simulink model "P702_NI_SoftECU"  (R2019a)
settings: Solver=ode1  StartTime=0.0  StopTime=Inf  FixedStep=0.001  RelTol=1e-3  EnableMultiTasking=on
PreLoadFcn:
  | run '.\VeriStand_BlockSet\NIVeriStandAddPaths.m'
undefined symbols (not defined in the file or in its folder): magnitude
libraries: simulink x83, simulink_extras x1
(part 71 of 76)

== system P702_NI_SoftECU/SoftECU/SRR_R/RearRight_SOD/SRR_RR_002/Subsystem ==
  target_pos : Inport
  sensor_pos : Inport  Port=2
  CSP : Inport  Port=3
  Abs : Abs
  Add : Sum  Inputs=++-+
  Add1 : Sum  Inputs=++-+
  Add2 : Sum  Inputs=+-
  Add3 : Sum
  Bus Selector : BusSelector  OutputSignals=SRR_R_DET_RANGE_02[m],SRR_R_DET_AZIMUTH_02[rad],SRR_R_DET_RANGE_RATE_02[m/s],SRR_R_DET_ELEVATION_02[rad]
  Bus Selector1 : BusSelector  OutputSignals=sensor_x,sensor_y,sensor_yaw
  Bus Selector2 : BusSelector  OutputSignals=c_sensor_x,c_sensor_y,c_sensor_yaw
  Constant : Constant
  Index Vector : MultiPortSwitch  DataPortOrder=Zero-based contiguous  Inputs=2  zeroidx=on
  Index Vector1 : MultiPortSwitch  DataPortOrder=Zero-based contiguous  Inputs=2  zeroidx=on
  Logical Operator : Logic  AllPortsSameDT=off  OutDataTypeStr=boolean
  Math Function : Math  Operator=magnitude^2  SaturateOnIntegerOverflow=on
  Math Function1 : Math  Operator=magnitude^2  SaturateOnIntegerOverflow=on
  Product : Product
  Product1 : Product
  Product2 : Product
  Relational Operator : RelationalOperator  Operator=<=  OutDataTypeStr=boolean  RndMeth=Simplest
  Relational Operator1 : RelationalOperator  Operator=<=  OutDataTypeStr=boolean  RndMeth=Simplest
  Sqrt : Sqrt  SaturateOnIntegerOverflow=on
  Terminator : Terminator
  atan_cal : Trigonometry  Operator=atan2
  atan_cal1 : Trigonometry  Operator=atan2
  not_valid_azimuth : Constant  Value=0
  not_valid_range : Constant  Value=-1
  random_factor : Subsystem
  random_factor1 : Subsystem
  sincal : Trigonometry
  sincal1 : Trigonometry  Operator=cos
  sincal2 : Trigonometry
  sincal3 : Trigonometry  Operator=cos
  range : Outport
  range_rate : Outport  Port=2
  azimuth : Outport  Port=3
  elevation : Outport  Port=4
  wires:
  random_factor1/1(Rand_Error) -> Add1/4
  random_factor/1(Rand_Error) -> Add/4
  [AngleScanRange] -> Relational Operator1/2
  [DistanceScanRange] -> Relational Operator/2
  Abs/1 -> Relational Operator1/1
  Add2/1 -> sincal2/1, sincal3/1
  sincal3/1 -> atan_cal1/2
  sincal2/1 -> atan_cal1/1
  atan_cal1/1 -> Product2/1
  not_valid_azimuth/1 -> Index Vector1/2
  Logical Operator/1 -> Index Vector/1, Index Vector1/1
  Index Vector1/1 -> azimuth/1
  not_valid_range/1 -> Index Vector/2
  Index Vector/1 -> range/1
  Relational Operator1/1 -> Logical Operator/2
  Relational Operator/1 -> Logical Operator/1
  Product2/1 -> Index Vector1/3, Abs/1
  Sqrt/1 -> Relational Operator/1, Index Vector/3
  Bus Selector/4 -> elevation/1  "<SRR_R_DET_ELEVATION_02[rad]>"
  Bus Selector/3 -> range_rate/1  "<SRR_R_DET_RANGE_RATE_02[m/s]>"
  Constant/1 -> Product2/2
  Add3/1 -> Sqrt/1
  Math Function1/1 -> Add3/2
  Math Function/1 -> Add3/1
  atan_cal/1 -> Add2/1
  Add1/1 -> atan_cal/2, Math Function1/1
  Add/1 -> atan_cal/1, Math Function/1
  Product1/1 -> Add1/1
  Bus Selector1/3 -> Add2/2  "<sensor_yaw>"
  Bus Selector1/2 -> Add/3  "<sensor_y>"
  Bus Selector1/1 -> Add1/3  "<sensor_x>"
  Bus Selector2/3 -> Terminator/1  "<c_sensor_yaw>"
  Bus Selector2/2 -> Add/2  "<c_sensor_y>"
  Bus Selector2/1 -> Add1/2  "<c_sensor_x>"
  CSP/1 -> Bus Selector2/1
  sensor_pos/1 -> Bus Selector1/1
  Product/1 -> Add/1
  sincal1/1 -> Product1/2
  sincal/1 -> Product/2
  Bus Selector/2 -> sincal/1, sincal1/1  "<SRR_R_DET_AZIMUTH_02[rad]>"
  Bus Selector/1 -> Product/1, Product1/1, random_factor1/1(Range), random_factor/1(Range)  "<SRR_R_DET_RANGE_02[m]>"
  target_pos/1 -> Bus Selector/1

== system P702_NI_SoftECU/SoftECU/SRR_R/RearRight_SOD/SRR_RR_003/Subsystem ==
  target_pos : Inport
  sensor_pos : Inport  Port=2
  CSP : Inport  Port=3
  Abs : Abs
  Add : Sum  Inputs=++-+
  Add1 : Sum  Inputs=++-+
  Add2 : Sum  Inputs=+-
  Add3 : Sum
  Bus Selector : BusSelector  OutputSignals=SRR_R_DET_RANGE_03[m],SRR_R_DET_AZIMUTH_03[rad],SRR_R_DET_RANGE_RATE_03[m/s],SRR_R_DET_ELEVATION_03[rad]
  Bus Selector1 : BusSelector  OutputSignals=sensor_x,sensor_y,sensor_yaw
  Bus Selector2 : BusSelector  OutputSignals=c_sensor_x,c_sensor_y,c_sensor_yaw
  Constant : Constant
  Index Vector : MultiPortSwitch  DataPortOrder=Zero-based contiguous  Inputs=2  zeroidx=on
  Index Vector1 : MultiPortSwitch  DataPortOrder=Zero-based contiguous  Inputs=2  zeroidx=on
  Logical Operator : Logic  AllPortsSameDT=off  OutDataTypeStr=boolean
  Math Function : Math  Operator=magnitude^2  SaturateOnIntegerOverflow=on
  Math Function1 : Math  Operator=magnitude^2  SaturateOnIntegerOverflow=on
  Product : Product
  Product1 : Product
  Product2 : Product
  Relational Operator : RelationalOperator  Operator=<=  OutDataTypeStr=boolean  RndMeth=Simplest
  Relational Operator1 : RelationalOperator  Operator=<=  OutDataTypeStr=boolean  RndMeth=Simplest
  Sqrt : Sqrt  SaturateOnIntegerOverflow=on
  Terminator : Terminator
  atan_cal : Trigonometry  Operator=atan2
  atan_cal1 : Trigonometry  Operator=atan2
  not_valid_azimuth : Constant  Value=0
  not_valid_range : Constant  Value=-1
  random_factor : Subsystem
  random_factor1 : Subsystem
  sincal : Trigonometry
  sincal1 : Trigonometry  Operator=cos
  sincal2 : Trigonometry
  sincal3 : Trigonometry  Operator=cos
  range : Outport
  range_rate : Outport  Port=2
  azimuth : Outport  Port=3
  elevation : Outport  Port=4
  wires:
  target_pos/1 -> Bus Selector/1
  Bus Selector/1 -> random_factor/1(Range), random_factor1/1(Range), Product1/1, Product/1  "<SRR_R_DET_RANGE_03[m]>"
  Bus Selector/2 -> sincal1/1, sincal/1  "<SRR_R_DET_AZIMUTH_03[rad]>"
  sincal/1 -> Product/2
  sincal1/1 -> Product1/2
  Product/1 -> Add/1
  sensor_pos/1 -> Bus Selector1/1
  CSP/1 -> Bus Selector2/1
  Bus Selector2/1 -> Add1/2  "<c_sensor_x>"
  Bus Selector2/2 -> Add/2  "<c_sensor_y>"
  Bus Selector2/3 -> Terminator/1  "<c_sensor_yaw>"
  Bus Selector1/1 -> Add1/3  "<sensor_x>"
  Bus Selector1/2 -> Add/3  "<sensor_y>"
  Bus Selector1/3 -> Add2/2  "<sensor_yaw>"
  Product1/1 -> Add1/1
  Add/1 -> Math Function/1, atan_cal/1
  Add1/1 -> Math Function1/1, atan_cal/2
  atan_cal/1 -> Add2/1
  Math Function/1 -> Add3/1
  Math Function1/1 -> Add3/2
  Add3/1 -> Sqrt/1
  Constant/1 -> Product2/2
  Bus Selector/3 -> range_rate/1  "<SRR_R_DET_RANGE_RATE_03[m/s]>"
  Bus Selector/4 -> elevation/1  "<SRR_R_DET_ELEVATION_03[rad]>"
  Sqrt/1 -> Index Vector/3, Relational Operator/1
  Product2/1 -> Abs/1, Index Vector1/3
  Relational Operator/1 -> Logical Operator/1
  Relational Operator1/1 -> Logical Operator/2
  Index Vector/1 -> range/1
  not_valid_range/1 -> Index Vector/2
  Index Vector1/1 -> azimuth/1
  Logical Operator/1 -> Index Vector1/1, Index Vector/1
  not_valid_azimuth/1 -> Index Vector1/2
  atan_cal1/1 -> Product2/1
  sincal2/1 -> atan_cal1/1
  sincal3/1 -> atan_cal1/2
  Add2/1 -> sincal3/1, sincal2/1
  Abs/1 -> Relational Operator1/1
  [DistanceScanRange] -> Relational Operator/2
  [AngleScanRange] -> Relational Operator1/2
  random_factor/1(Rand_Error) -> Add/4
  random_factor1/1(Rand_Error) -> Add1/4

== system P702_NI_SoftECU/Output/Subsystem1/CAN_Signal/GWM/GSM/Gear_Shift_by_Wire_2_FD1_168 ==
  in_port : Inport
  GearButtnStuck_B_Actl : Terminator
  GsmSrvcRqd_B_Rq : Terminator
  TrnGearPwmFalt_B_Actl : Terminator
  TrnTrcmPwmSig_D_Actl : Terminator
  bus_selector : BusSelector  OutputSignals=GearButtnStuck_B_Actl,GsmSrvcRqd_B_Rq,TrnGearPwmFalt_B_Actl,TrnTrcmPwmSig_D_Actl
  wires:
  in_port/1 -> bus_selector/1  "Subsystem1"
  bus_selector/1 -> GearButtnStuck_B_Actl/1  "<GearButtnStuck_B_Actl>"
  bus_selector/2 -> GsmSrvcRqd_B_Rq/1  "<GsmSrvcRqd_B_Rq>"
  bus_selector/3 -> TrnGearPwmFalt_B_Actl/1  "<TrnGearPwmFalt_B_Actl>"
  bus_selector/4 -> TrnTrcmPwmSig_D_Actl/1  "<TrnTrcmPwmSig_D_Actl>"

== system P702_NI_SoftECU/Output/Subsystem1/CAN_Signal/GWM/GSM/Gear_Shift_by_Wire_FD1_5A ==
  in_port : Inport
  BrkSwtchPos_B_ActlGsm : Terminator
  DrQltyDrv_D_StatGsm : Terminator
  GsmGearMsgTxt_D_Rq : Terminator
  PrkBrkActv_D_RqGsmGear : Terminator
  TrnBtsiOvrrd_B_Stat : Terminator
  TrnGearButtn_B_ActlD0 : Terminator
  TrnGearButtn_B_ActlD1 : Terminator
  TrnGearButtn_B_ActlD2 : Terminator
  TrnGearButtn_B_ActlM0 : Terminator
  TrnGearButtn_B_ActlM1 : Terminator
  TrnGearButtn_B_ActlM2 : Terminator
  TrnGearButtn_B_ActlN0 : Terminator
  TrnGearButtn_B_ActlN1 : Terminator
  TrnGearButtn_B_ActlN2 : Terminator
  TrnGearButtn_B_ActlP0 : Terminator
  TrnGearButtn_B_ActlP1 : Terminator
  TrnGearButtn_B_ActlP2 : Terminator
  TrnGearButtn_B_ActlR0 : Terminator
  TrnGearButtn_B_ActlR1 : Terminator
  TrnGearButtn_B_ActlR2 : Terminator
  TrnGearButtn_U_Actl : Terminator
  TrnGearRqCnt_B_Actl : Terminator
  TrnGear_D_RqDrv : Terminator
  TrnGear_No_Cnt : Terminator
  TrnGear_No_Cs : Terminator
  TrnGsmNtmState_D_Actl : Terminator
  TrnRng_D_RqGsm : Terminator
  TrnValidGearRq_D_Stat : Terminator
  bus_selector : BusSelector  OutputSignals=BrkSwtchPos_B_ActlGsm,DrQltyDrv_D_StatGsm,GsmGearMsgTxt_D_Rq,PrkBrkActv_D_RqGsmGear,TrnBtsiOvrrd_B_Stat,TrnGearButtn_B_ActlD0,TrnGearButtn_B_ActlD1,TrnGearButtn_B_ActlD2,TrnGearButtn_B_ActlM0,TrnGearButtn_B_ActlM1,TrnGearButtn_B_ActlM2,TrnGearButtn_B_ActlN0,TrnGearButtn_B_ActlN1,TrnGearButtn_B_ActlN2,TrnGearButtn_B_ActlP0,TrnGearButtn_B_ActlP1,TrnGearButtn_B_ActlP2,TrnGearButtn_B_ActlR0,TrnGearButtn_B_ActlR1,TrnGearButtn_B_ActlR2,TrnGearButtn_U_Actl,TrnGearRqCnt_B_Actl,TrnGear_D_RqDrv,TrnGear_No_Cnt,TrnGear_No_Cs,TrnGsmNtmState_D_Actl,TrnRng_D_RqGsm,TrnValidGearRq_D_Stat
  wires:
  in_port/1 -> bus_selector/1  "Subsystem1"
  bus_selector/1 -> BrkSwtchPos_B_ActlGsm/1  "<BrkSwtchPos_B_ActlGsm>"
  bus_selector/2 -> DrQltyDrv_D_StatGsm/1  "<DrQltyDrv_D_StatGsm>"
  bus_selector/3 -> GsmGearMsgTxt_D_Rq/1  "<GsmGearMsgTxt_D_Rq>"
  bus_selector/4 -> PrkBrkActv_D_RqGsmGear/1  "<PrkBrkActv_D_RqGsmGear>"
  bus_selector/5 -> TrnBtsiOvrrd_B_Stat/1  "<TrnBtsiOvrrd_B_Stat>"
  bus_selector/6 -> TrnGearButtn_B_ActlD0/1  "<TrnGearButtn_B_ActlD0>"
  bus_selector/7 -> TrnGearButtn_B_ActlD1/1  "<TrnGearButtn_B_ActlD1>"
  bus_selector/8 -> TrnGearButtn_B_ActlD2/1  "<TrnGearButtn_B_ActlD2>"
  bus_selector/9 -> TrnGearButtn_B_ActlM0/1  "<TrnGearButtn_B_ActlM0>"
  bus_selector/10 -> TrnGearButtn_B_ActlM1/1  "<TrnGearButtn_B_ActlM1>"
  bus_selector/11 -> TrnGearButtn_B_ActlM2/1  "<TrnGearButtn_B_ActlM2>"
  bus_selector/12 -> TrnGearButtn_B_ActlN0/1  "<TrnGearButtn_B_ActlN0>"
  bus_selector/13 -> TrnGearButtn_B_ActlN1/1  "<TrnGearButtn_B_ActlN1>"
  bus_selector/14 -> TrnGearButtn_B_ActlN2/1  "<TrnGearButtn_B_ActlN2>"
  bus_selector/15 -> TrnGearButtn_B_ActlP0/1  "<TrnGearButtn_B_ActlP0>"
  bus_selector/16 -> TrnGearButtn_B_ActlP1/1  "<TrnGearButtn_B_ActlP1>"
  bus_selector/17 -> TrnGearButtn_B_ActlP2/1  "<TrnGearButtn_B_ActlP2>"
  bus_selector/18 -> TrnGearButtn_B_ActlR0/1  "<TrnGearButtn_B_ActlR0>"
  bus_selector/19 -> TrnGearButtn_B_ActlR1/1  "<TrnGearButtn_B_ActlR1>"
  bus_selector/20 -> TrnGearButtn_B_ActlR2/1  "<TrnGearButtn_B_ActlR2>"
  bus_selector/21 -> TrnGearButtn_U_Actl/1  "<TrnGearButtn_U_Actl>"
  bus_selector/22 -> TrnGearRqCnt_B_Actl/1  "<TrnGearRqCnt_B_Actl>"
  bus_selector/23 -> TrnGear_D_RqDrv/1  "<TrnGear_D_RqDrv>"
  bus_selector/24 -> TrnGear_No_Cnt/1  "<TrnGear_No_Cnt>"
  bus_selector/25 -> TrnGear_No_Cs/1  "<TrnGear_No_Cs>"
  bus_selector/26 -> TrnGsmNtmState_D_Actl/1  "<TrnGsmNtmState_D_Actl>"
  bus_selector/27 -> TrnRng_D_RqGsm/1  "<TrnRng_D_RqGsm>"
  bus_selector/28 -> TrnValidGearRq_D_Stat/1  "<TrnValidGearRq_D_Stat>"

== system P702_NI_SoftECU/Output/Subsystem1/CAN_Signal/GWM/Other_GWMTx/AC_Compressor_Data_FD1 ==
  in_port : Inport
  ElCmprBattSysU_D_Falt : Terminator
  ElCmprBattURng_D_Falt : Terminator
  ElCmprInnrErr_D_Falt : Terminator
  ElCmprLostComm_D_Falt : Terminator
  ElCmprOverLoad_D_Falt : Terminator
  ElCmprOverTe_D_Falt : Terminator
  ElCmprOverTe_D_Stat : Terminator
  ElCmprPerfErr_D_Falt : Terminator
  ElCmprSysU_D_Falt : Terminator
  ElCmprUHi_D_Stat : Terminator
  ElCmprUHi_U_Actl : Terminator
  ElCmpr_D_Stat : Terminator
  ElCmpr_N_Actl : Terminator
  ElCmpr_Pw_Actl : Terminator
  bus_selector : BusSelector  OutputSignals=ElCmprBattSysU_D_Falt,ElCmprBattURng_D_Falt,ElCmprInnrErr_D_Falt,ElCmprLostComm_D_Falt,ElCmprOverLoad_D_Falt,ElCmprOverTe_D_Falt,ElCmprOverTe_D_Stat,ElCmprPerfErr_D_Falt,ElCmprSysU_D_Falt,ElCmprUHi_D_Stat,ElCmprUHi_U_Actl,ElCmpr_D_Stat,ElCmpr_N_Actl,ElCmpr_Pw_Actl
  wires:
  in_port/1 -> bus_selector/1  "Subsystem1"
  bus_selector/1 -> ElCmprBattSysU_D_Falt/1  "<ElCmprBattSysU_D_Falt>"
  bus_selector/2 -> ElCmprBattURng_D_Falt/1  "<ElCmprBattURng_D_Falt>"
  bus_selector/3 -> ElCmprInnrErr_D_Falt/1  "<ElCmprInnrErr_D_Falt>"
  bus_selector/4 -> ElCmprLostComm_D_Falt/1  "<ElCmprLostComm_D_Falt>"
  bus_selector/5 -> ElCmprOverLoad_D_Falt/1  "<ElCmprOverLoad_D_Falt>"
  bus_selector/6 -> ElCmprOverTe_D_Falt/1  "<ElCmprOverTe_D_Falt>"
  bus_selector/7 -> ElCmprOverTe_D_Stat/1  "<ElCmprOverTe_D_Stat>"
  bus_selector/8 -> ElCmprPerfErr_D_Falt/1  "<ElCmprPerfErr_D_Falt>"
  bus_selector/9 -> ElCmprSysU_D_Falt/1  "<ElCmprSysU_D_Falt>"
  bus_selector/10 -> ElCmprUHi_D_Stat/1  "<ElCmprUHi_D_Stat>"
  bus_selector/11 -> ElCmprUHi_U_Actl/1  "<ElCmprUHi_U_Actl>"
  bus_selector/12 -> ElCmpr_D_Stat/1  "<ElCmpr_D_Stat>"
  bus_selector/13 -> ElCmpr_N_Actl/1  "<ElCmpr_N_Actl>"
  bus_selector/14 -> ElCmpr_Pw_Actl/1  "<ElCmpr_Pw_Actl>"

== system P702_NI_SoftECU/Output/Subsystem1/CAN_Signal/GWM/Other_GWMTx/AC_Compressor_Req_FD1 ==
  in_port : Inport
  ElCmprEnbl_B_Rq : Terminator
  ElCmpr_N_Rq : Terminator
  bus_selector : BusSelector  OutputSignals=ElCmprEnbl_B_Rq,ElCmpr_N_Rq
  wires:
  in_port/1 -> bus_selector/1  "Subsystem1"
  bus_selector/1 -> ElCmprEnbl_B_Rq/1  "<ElCmprEnbl_B_Rq>"
  bus_selector/2 -> ElCmpr_N_Rq/1  "<ElCmpr_N_Rq>"

== system P702_NI_SoftECU/Output/Subsystem1/CAN_Signal/GWM/Other_GWMTx/APIMGPS_Data_Nav_1_FD1 ==
  in_port : Inport
  GPS_Latitude_Degrees : Terminator
  GPS_Latitude_Min_dec : Terminator
  GPS_Latitude_Minutes : Terminator
  GPS_Longitude_Degrees : Terminator
  GPS_Longitude_Min_dec : Terminator
  GPS_Longitude_Minutes : Terminator
  GpsHsphLattSth_D_Actl : Terminator
  GpsHsphLongEast_D_Actl : Terminator
  bus_selector : BusSelector  OutputSignals=GPS_Latitude_Degrees,GPS_Latitude_Min_dec,GPS_Latitude_Minutes,GPS_Longitude_Degrees,GPS_Longitude_Min_dec,GPS_Longitude_Minutes,GpsHsphLattSth_D_Actl,GpsHsphLongEast_D_Actl
  wires:
  in_port/1 -> bus_selector/1  "Subsystem1"
  bus_selector/1 -> GPS_Latitude_Degrees/1  "<GPS_Latitude_Degrees>"
  bus_selector/2 -> GPS_Latitude_Min_dec/1  "<GPS_Latitude_Min_dec>"
  bus_selector/3 -> GPS_Latitude_Minutes/1  "<GPS_Latitude_Minutes>"
  bus_selector/4 -> GPS_Longitude_Degrees/1  "<GPS_Longitude_Degrees>"
  bus_selector/5 -> GPS_Longitude_Min_dec/1  "<GPS_Longitude_Min_dec>"
  bus_selector/6 -> GPS_Longitude_Minutes/1  "<GPS_Longitude_Minutes>"
  bus_selector/7 -> GpsHsphLattSth_D_Actl/1  "<GpsHsphLattSth_D_Actl>"
  bus_selector/8 -> GpsHsphLongEast_D_Actl/1  "<GpsHsphLongEast_D_Actl>"

== system P702_NI_SoftECU/Output/Subsystem1/CAN_Signal/GWM/Other_GWMTx/APIMGPS_Data_Nav_2_FD1 ==
  in_port : Inport
  GPS_Actual_vs_Infer_pos : Terminator
  GPS_Compass_direction : Terminator
  GPS_Pdop : Terminator
  GPS_UTC_hours : Terminator
  GPS_UTC_minutes : Terminator
  GPS_UTC_seconds : Terminator
  GpsUtcDay_No_Actl : Terminator
  GpsUtcMnth_No_Actl : Terminator
  GpsUtcYr_No_Actl : Terminator
  Gps_B_Falt : Terminator
  bus_selector : BusSelector  OutputSignals=GPS_Actual_vs_Infer_pos,GPS_Compass_direction,GPS_Pdop,GPS_UTC_hours,GPS_UTC_minutes,GPS_UTC_seconds,GpsUtcDay_No_Actl,GpsUtcMnth_No_Actl,GpsUtcYr_No_Actl,Gps_B_Falt
  wires:
  in_port/1 -> bus_selector/1  "Subsystem1"
  bus_selector/1 -> GPS_Actual_vs_Infer_pos/1  "<GPS_Actual_vs_Infer_pos>"
  bus_selector/2 -> GPS_Compass_direction/1  "<GPS_Compass_direction>"
  bus_selector/3 -> GPS_Pdop/1  "<GPS_Pdop>"
  bus_selector/4 -> GPS_UTC_hours/1  "<GPS_UTC_hours>"
  bus_selector/5 -> GPS_UTC_minutes/1  "<GPS_UTC_minutes>"
  bus_selector/6 -> GPS_UTC_seconds/1  "<GPS_UTC_seconds>"
  bus_selector/7 -> GpsUtcDay_No_Actl/1  "<GpsUtcDay_No_Actl>"
  bus_selector/8 -> GpsUtcMnth_No_Actl/1  "<GpsUtcMnth_No_Actl>"
  bus_selector/9 -> GpsUtcYr_No_Actl/1  "<GpsUtcYr_No_Actl>"
  bus_selector/10 -> Gps_B_Falt/1  "<Gps_B_Falt>"

== system P702_NI_SoftECU/Output/Subsystem1/CAN_Signal/GWM/Other_GWMTx/APIM_Request_Signals_1_FD1 ==
  in_port : Inport
  ChrgOvrdExitScrn_D_Rq : Terminator
  EmPrflButtnAssoc_D_Rq : Terminator
  EmPrflKeyAssoc_D_Rq : Terminator
  EmPrflNo_D_Rq : Terminator
  Em_D_Stat : Terminator
  Rba_D_Rq : Terminator
  bus_selector : BusSelector  OutputSignals=ChrgOvrdExitScrn_D_Rq,EmPrflButtnAssoc_D_Rq,EmPrflKeyAssoc_D_Rq,EmPrflNo_D_Rq,Em_D_Stat,Rba_D_Rq
  wires:
  in_port/1 -> bus_selector/1  "Subsystem1"
  bus_selector/1 -> ChrgOvrdExitScrn_D_Rq/1  "<ChrgOvrdExitScrn_D_Rq>"
  bus_selector/2 -> EmPrflButtnAssoc_D_Rq/1  "<EmPrflButtnAssoc_D_Rq>"
  bus_selector/3 -> EmPrflKeyAssoc_D_Rq/1  "<EmPrflKeyAssoc_D_Rq>"
  bus_selector/4 -> EmPrflNo_D_Rq/1  "<EmPrflNo_D_Rq>"
  bus_selector/5 -> Em_D_Stat/1  "<Em_D_Stat>"
  bus_selector/6 -> Rba_D_Rq/1  "<Rba_D_Rq>"

== system P702_NI_SoftECU/Output/Subsystem1/CAN_Signal/GWM/Other_GWMTx/APIM_Request_Signals_FD1 ==
  in_port : Inport
  CbnCmrtPrefListIndx_Rq : Terminator
  CbnCmrtPrefLstNmItm_Rq : Terminator
  ChargePortPwr_Rq : Terminator
  ChrgStatDsply_D_Rq : Terminator
  FactoryReset_Rq : Terminator
  LongTermParking_Rq : Terminator
  ModemReset_D_Rq : Terminator
  NextUsageTimeToggle_Rq : Terminator
  OffPeakTimeSetHR_Rq : Terminator
  OffPeakTimeSetMin_Rq : Terminator
  StopStrtDrvMde_B_RqBtn3 : Terminator
  TCU_ESN_D_Rq : Terminator
  bus_selector : BusSelector  OutputSignals=CbnCmrtPrefListIndx_Rq,CbnCmrtPrefLstNmItm_Rq,ChargePortPwr_Rq,ChrgStatDsply_D_Rq,FactoryReset_Rq,LongTermParking_Rq,ModemReset_D_Rq,NextUsageTimeToggle_Rq,OffPeakTimeSetHR_Rq,OffPeakTimeSetMin_Rq,StopStrtDrvMde_B_RqBtn3,TCU_ESN_D_Rq
  wires:
  in_port/1 -> bus_selector/1  "Subsystem1"
  bus_selector/1 -> CbnCmrtPrefListIndx_Rq/1  "<CbnCmrtPrefListIndx_Rq>"
  bus_selector/2 -> CbnCmrtPrefLstNmItm_Rq/1  "<CbnCmrtPrefLstNmItm_Rq>"
  bus_selector/3 -> ChargePortPwr_Rq/1  "<ChargePortPwr_Rq>"
  bus_selector/4 -> ChrgStatDsply_D_Rq/1  "<ChrgStatDsply_D_Rq>"
  bus_selector/5 -> FactoryReset_Rq/1  "<FactoryReset_Rq>"
  bus_selector/6 -> LongTermParking_Rq/1  "<LongTermParking_Rq>"
  bus_selector/7 -> ModemReset_D_Rq/1  "<ModemReset_D_Rq>"
  bus_selector/8 -> NextUsageTimeToggle_Rq/1  "<NextUsageTimeToggle_Rq>"
  bus_selector/9 -> OffPeakTimeSetHR_Rq/1  "<OffPeakTimeSetHR_Rq>"
  bus_selector/10 -> OffPeakTimeSetMin_Rq/1  "<OffPeakTimeSetMin_Rq>"
  bus_selector/11 -> StopStrtDrvMde_B_RqBtn3/1  "<StopStrtDrvMde_B_RqBtn3>"
  bus_selector/12 -> TCU_ESN_D_Rq/1  "<TCU_ESN_D_Rq>"

== system P702_NI_SoftECU/Output/Subsystem1/CAN_Signal/GWM/Other_GWMTx/APIM_Send_Signals1_FD1 ==
  in_port : Inport
  APIM_ActiveTrackNum_St : Terminator
  APIM_NumberofTracks_St : Terminator
  AutoHoldSwtch_D_Stat3 : Terminator
  CenterStackRing_D_Actl : Terminator
  ChrgCordUnlock_B_Rq : Terminator
  TrlrAidCancl_B_Rq : Terminator
  TrlrAidSetup_D_Stat : Terminator
  TrlrTrgtAcquire_D_Rq : Terminator
  ValetMode_D_Stat : Terminator
  bus_selector : BusSelector  OutputSignals=APIM_ActiveTrackNum_St,APIM_NumberofTracks_St,AutoHoldSwtch_D_Stat3,CenterStackRing_D_Actl,ChrgCordUnlock_B_Rq,TrlrAidCancl_B_Rq,TrlrAidSetup_D_Stat,TrlrTrgtAcquire_D_Rq,ValetMode_D_Stat
  wires:
  in_port/1 -> bus_selector/1  "Subsystem1"
  bus_selector/1 -> APIM_ActiveTrackNum_St/1  "<APIM_ActiveTrackNum_St>"
  bus_selector/2 -> APIM_NumberofTracks_St/1  "<APIM_NumberofTracks_St>"
  bus_selector/3 -> AutoHoldSwtch_D_Stat3/1  "<AutoHoldSwtch_D_Stat3>"
  bus_selector/4 -> CenterStackRing_D_Actl/1  "<CenterStackRing_D_Actl>"
  bus_selector/5 -> ChrgCordUnlock_B_Rq/1  "<ChrgCordUnlock_B_Rq>"
  bus_selector/6 -> TrlrAidCancl_B_Rq/1  "<TrlrAidCancl_B_Rq>"
  bus_selector/7 -> TrlrAidSetup_D_Stat/1  "<TrlrAidSetup_D_Stat>"
  bus_selector/8 -> TrlrTrgtAcquire_D_Rq/1  "<TrlrTrgtAcquire_D_Rq>"
  bus_selector/9 -> ValetMode_D_Stat/1  "<ValetMode_D_Stat>"

== system P702_NI_SoftECU/Output/Subsystem1/CAN_Signal/GWM/Other_GWMTx/APIM_Send_Signals_2_FD1 ==
  in_port : Inport
  OnbChrgClearAll_B_Rq : Terminator
  OnbChrgGoTDelete_B_Rq : Terminator
  OnbChrgGoTElement_D_Rq : Terminator
  OnbChrgGoTExtHtr_D_Rq : Terminator
  OnbChrgGoTHr_T_Rq : Terminator
  OnbChrgGoTMnte_D_Rq : Terminator
  OnbChrgGoTOn_D_Rq : Terminator
  OnbChrgGoTPrcond_D_Rq : Terminator
  OnbChrgGoTTouch_D_Rq : Terminator
  OnbChrgGoTUpdate_B_Rq : Terminator
  OtaTrg_D_Stat : Terminator
  PaakMyKey_D_Rq : Terminator
  TCU_Final_Actvtn_St : Terminator
  TCU_Init_Actvtn_St : Terminator
  TrlrAidMde_D_Rq : Terminator
  bus_selector : BusSelector  OutputSignals=OnbChrgClearAll_B_Rq,OnbChrgGoTDelete_B_Rq,OnbChrgGoTElement_D_Rq,OnbChrgGoTExtHtr_D_Rq,OnbChrgGoTHr_T_Rq,OnbChrgGoTMnte_D_Rq,OnbChrgGoTOn_D_Rq,OnbChrgGoTPrcond_D_Rq,OnbChrgGoTTouch_D_Rq,OnbChrgGoTUpdate_B_Rq,OtaTrg_D_Stat,PaakMyKey_D_Rq,TCU_Final_Actvtn_St,TCU_Init_Actvtn_St,TrlrAidMde_D_Rq
  wires:
  in_port/1 -> bus_selector/1  "Subsystem1"
  bus_selector/1 -> OnbChrgClearAll_B_Rq/1  "<OnbChrgClearAll_B_Rq>"
  bus_selector/2 -> OnbChrgGoTDelete_B_Rq/1  "<OnbChrgGoTDelete_B_Rq>"
  bus_selector/3 -> OnbChrgGoTElement_D_Rq/1  "<OnbChrgGoTElement_D_Rq>"
  bus_selector/4 -> OnbChrgGoTExtHtr_D_Rq/1  "<OnbChrgGoTExtHtr_D_Rq>"
  bus_selector/5 -> OnbChrgGoTHr_T_Rq/1  "<OnbChrgGoTHr_T_Rq>"
  bus_selector/6 -> OnbChrgGoTMnte_D_Rq/1  "<OnbChrgGoTMnte_D_Rq>"
  bus_selector/7 -> OnbChrgGoTOn_D_Rq/1  "<OnbChrgGoTOn_D_Rq>"
  bus_selector/8 -> OnbChrgGoTPrcond_D_Rq/1  "<OnbChrgGoTPrcond_D_Rq>"
  bus_selector/9 -> OnbChrgGoTTouch_D_Rq/1  "<OnbChrgGoTTouch_D_Rq>"
  bus_selector/10 -> OnbChrgGoTUpdate_B_Rq/1  "<OnbChrgGoTUpdate_B_Rq>"
  bus_selector/11 -> OtaTrg_D_Stat/1  "<OtaTrg_D_Stat>"
  bus_selector/12 -> PaakMyKey_D_Rq/1  "<PaakMyKey_D_Rq>"
  bus_selector/13 -> TCU_Final_Actvtn_St/1  "<TCU_Final_Actvtn_St>"
  bus_selector/14 -> TCU_Init_Actvtn_St/1  "<TCU_Init_Actvtn_St>"
  bus_selector/15 -> TrlrAidMde_D_Rq/1  "<TrlrAidMde_D_Rq>"

== system P702_NI_SoftECU/Output/Subsystem1/CAN_Signal/GWM/Other_GWMTx/ActiveFrontStrg_Stat2_FD1 ==
  in_port : Inport
  SteWhlRelCalib_An_Sns : Terminator
  SteWhlRelCalib_T_Actl : Terminator
  bus_selector : BusSelector  OutputSignals=SteWhlRelCalib_An_Sns,SteWhlRelCalib_T_Actl
  wires:
  in_port/1 -> bus_selector/1  "Subsystem1"
  bus_selector/1 -> SteWhlRelCalib_An_Sns/1  "<SteWhlRelCalib_An_Sns>"
  bus_selector/2 -> SteWhlRelCalib_T_Actl/1  "<SteWhlRelCalib_T_Actl>"

== system P702_NI_SoftECU/Output/Subsystem1/CAN_Signal/GWM/Other_GWMTx/ActiveFrontStrg_Stat_FD1 ==
  in_port : Inport
  SteWhlBrkAnActl_No_Cnt : Terminator
  SteWhlBrkAnActl_No_Cs : Terminator
  SteWhlBrkOffst_An_Actl : Terminator
  SteWhlOffstRq_D_Stat : Terminator
  SteWhlOffst_An_TotActl : Terminator
  bus_selector : BusSelector  OutputSignals=SteWhlBrkAnActl_No_Cnt,SteWhlBrkAnActl_No_Cs,SteWhlBrkOffst_An_Actl,SteWhlOffstRq_D_Stat,SteWhlOffst_An_TotActl
  wires:
  in_port/1 -> bus_selector/1  "Subsystem1"
  bus_selector/1 -> SteWhlBrkAnActl_No_Cnt/1  "<SteWhlBrkAnActl_No_Cnt>"
  bus_selector/2 -> SteWhlBrkAnActl_No_Cs/1  "<SteWhlBrkAnActl_No_Cs>"
  bus_selector/3 -> SteWhlBrkOffst_An_Actl/1  "<SteWhlBrkOffst_An_Actl>"
  bus_selector/4 -> SteWhlOffstRq_D_Stat/1  "<SteWhlOffstRq_D_Stat>"
  bus_selector/5 -> SteWhlOffst_An_TotActl/1  "<SteWhlOffst_An_TotActl>"

== system P702_NI_SoftECU/Output/Subsystem1/CAN_Signal/GWM/Other_GWMTx/AllTerrainControlData_FD1 ==
  in_port : Inport
  SelDrvMdeCnt_D_Stat : Terminator
  SelDrvMdeSwtchOk_D_Stat : Terminator
  SelDrvMdeSwtch_D_Stat : Terminator
  SelDrvMdeSwtch_No_Actl : Terminator
  bus_selector : BusSelector  OutputSignals=SelDrvMdeCnt_D_Stat,SelDrvMdeSwtchOk_D_Stat,SelDrvMdeSwtch_D_Stat,SelDrvMdeSwtch_No_Actl
  wires:
  in_port/1 -> bus_selector/1  "Subsystem1"
  bus_selector/1 -> SelDrvMdeCnt_D_Stat/1  "<SelDrvMdeCnt_D_Stat>"
  bus_selector/2 -> SelDrvMdeSwtchOk_D_Stat/1  "<SelDrvMdeSwtchOk_D_Stat>"
  bus_selector/3 -> SelDrvMdeSwtch_D_Stat/1  "<SelDrvMdeSwtch_D_Stat>"
  bus_selector/4 -> SelDrvMdeSwtch_No_Actl/1  "<SelDrvMdeSwtch_No_Actl>"

== system P702_NI_SoftECU/Output/Subsystem1/CAN_Signal/GWM/Other_GWMTx/All_Terrain_Data_FD1 ==
  in_port : Inport
  TerrMde_D_RqDrv : Terminator
  TerrStat_D_RqDsply : Terminator
  bus_selector : BusSelector  OutputSignals=TerrMde_D_RqDrv,TerrStat_D_RqDsply
  wires:
  in_port/1 -> bus_selector/1  "Subsystem1"
  bus_selector/1 -> TerrMde_D_RqDrv/1  "<TerrMde_D_RqDrv>"
  bus_selector/2 -> TerrStat_D_RqDsply/1  "<TerrStat_D_RqDsply>"

== system P702_NI_SoftECU/Output/Subsystem1/CAN_Signal/GWM/Other_GWMTx/BCM_Lamp_Stat_FD1 ==
  in_port : Inport
  BrkWarnInd_B_Rq : Terminator
  Brk_Fluid_Lvl_Low : Terminator
  Courtesy_BSave_Stat : Terminator
  Courtesy_Delay_Status : Terminator
  CrnrLghtLeft_Pc_Rq : Terminator
  CrnrLghtRight_Pc_Rq : Terminator
  DayRnngLampOn_B_Stat : Terminator
  DrTgateLck_D_Stat : Terminator
  Dr_Courtesy_Light_Stat : Terminator
  HeadLampLoActv_B_Stat : Terminator
  HeadLampLoFlOn_B_Stat : Terminator
  HeadLampLoFrOn_B_Stat : Terminator
  HeadLampLoOut_B_Stat : Terminator
  HeadLghtHiFdbck_D_Stat : Terminator
  HeadLghtHiOn_B_Stat : Terminator
  HeadLghtSwtch_D_Stat : Terminator
  Headlamp_On_Wrning_Cmd : Terminator
  HomeSafeLtChime_B_Rq : Terminator
  Illuminated_Entry_Stat : Terminator
  ImpactEvntFdbck_D_Stat : Terminator
  KeyInIgnWarn_B_Cmd : Terminator
  Park_Brake_Chime_Rqst : Terminator
  PerimeterAlarmChimeRq : Terminator
  Perimeter_Alarm_Status : Terminator
  PrkLght_D_Stat : Terminator
  PrkLightChime_B_Rq : Terminator
  PudLampDrv_D_Rq : Terminator
  PudLampPsngr_D_Rq : Terminator
  PudLamp_D_Rq : Terminator
  ReducedGuard_D_Stat : Terminator
  RvrseLghtOn_B_Stat : Terminator
  StopLghtOn_B_Stat : Terminator
  TrnNotInPrkChime_B_Rq : Terminator
  WndwGlbl_D_Cmd : Terminator
  WrlssAcsyChrgInhbt_B_Rq : Terminator
  bus_selector : BusSelector  OutputSignals=BrkWarnInd_B_Rq,Brk_Fluid_Lvl_Low,Courtesy_BSave_Stat,Courtesy_Delay_Status,CrnrLghtLeft_Pc_Rq,CrnrLghtRight_Pc_Rq,DayRnngLampOn_B_Stat,DrTgateLck_D_Stat,Dr_Courtesy_Light_Stat,HeadLampLoActv_B_Stat,HeadLampLoFlOn_B_Stat,HeadLampLoFrOn_B_Stat,HeadLampLoOut_B_Stat,HeadLghtHiFdbck_D_Stat,HeadLghtHiOn_B_Stat,HeadLghtSwtch_D_Stat,Headlamp_On_Wrning_Cmd,HomeSafeLtChime_B_Rq,Illuminated_Entry_Stat,ImpactEvntFdbck_D_Stat,KeyInIgnWarn_B_Cmd,Park_Brake_Chime_Rqst,PerimeterAlarmChimeRq,Perimeter_Alarm_Status,PrkLght_D_Stat,PrkLightChime_B_Rq,PudLampDrv_D_Rq,PudLampPsngr_D_Rq,PudLamp_D_Rq,ReducedGuard_D_Stat,RvrseLghtOn_B_Stat,StopLghtOn_B_Stat,TrnNotInPrkChime_B_Rq,WndwGlbl_D_Cmd,WrlssAcsyChrgInhbt_B_Rq
  wires:
  in_port/1 -> bus_selector/1  "Subsystem1"
  bus_selector/1 -> BrkWarnInd_B_Rq/1  "<BrkWarnInd_B_Rq>"
  bus_selector/2 -> Brk_Fluid_Lvl_Low/1  "<Brk_Fluid_Lvl_Low>"
  bus_selector/3 -> Courtesy_BSave_Stat/1  "<Courtesy_BSave_Stat>"
  bus_selector/4 -> Courtesy_Delay_Status/1  "<Courtesy_Delay_Status>"
  bus_selector/5 -> CrnrLghtLeft_Pc_Rq/1  "<CrnrLghtLeft_Pc_Rq>"
  bus_selector/6 -> CrnrLghtRight_Pc_Rq/1  "<CrnrLghtRight_Pc_Rq>"
  bus_selector/7 -> DayRnngLampOn_B_Stat/1  "<DayRnngLampOn_B_Stat>"
  bus_selector/8 -> DrTgateLck_D_Stat/1  "<DrTgateLck_D_Stat>"
  bus_selector/9 -> Dr_Courtesy_Light_Stat/1  "<Dr_Courtesy_Light_Stat>"
  bus_selector/10 -> HeadLampLoActv_B_Stat/1  "<HeadLampLoActv_B_Stat>"
  bus_selector/11 -> HeadLampLoFlOn_B_Stat/1  "<HeadLampLoFlOn_B_Stat>"
  bus_selector/12 -> HeadLampLoFrOn_B_Stat/1  "<HeadLampLoFrOn_B_Stat>"
  bus_selector/13 -> HeadLampLoOut_B_Stat/1  "<HeadLampLoOut_B_Stat>"
  bus_selector/14 -> HeadLghtHiFdbck_D_Stat/1  "<HeadLghtHiFdbck_D_Stat>"
  bus_selector/15 -> HeadLghtHiOn_B_Stat/1  "<HeadLghtHiOn_B_Stat>"
  bus_selector/16 -> HeadLghtSwtch_D_Stat/1  "<HeadLghtSwtch_D_Stat>"
  bus_selector/17 -> Headlamp_On_Wrning_Cmd/1  "<Headlamp_On_Wrning_Cmd>"
  bus_selector/18 -> HomeSafeLtChime_B_Rq/1  "<HomeSafeLtChime_B_Rq>"
  bus_selector/19 -> Illuminated_Entry_Stat/1  "<Illuminated_Entry_Stat>"
  bus_selector/20 -> ImpactEvntFdbck_D_Stat/1  "<ImpactEvntFdbck_D_Stat>"
  bus_selector/21 -> KeyInIgnWarn_B_Cmd/1  "<KeyInIgnWarn_B_Cmd>"
  bus_selector/22 -> Park_Brake_Chime_Rqst/1  "<Park_Brake_Chime_Rqst>"
  bus_selector/23 -> PerimeterAlarmChimeRq/1  "<PerimeterAlarmChimeRq>"
  bus_selector/24 -> Perimeter_Alarm_Status/1  "<Perimeter_Alarm_Status>"
  bus_selector/25 -> PrkLght_D_Stat/1  "<PrkLght_D_Stat>"
  bus_selector/26 -> PrkLightChime_B_Rq/1  "<PrkLightChime_B_Rq>"
  bus_selector/27 -> PudLampDrv_D_Rq/1  "<PudLampDrv_D_Rq>"
  bus_selector/28 -> PudLampPsngr_D_Rq/1  "<PudLampPsngr_D_Rq>"
  bus_selector/29 -> PudLamp_D_Rq/1  "<PudLamp_D_Rq>"
  bus_selector/30 -> ReducedGuard_D_Stat/1  "<ReducedGuard_D_Stat>"
  bus_selector/31 -> RvrseLghtOn_B_Stat/1  "<RvrseLghtOn_B_Stat>"
  bus_selector/32 -> StopLghtOn_B_Stat/1  "<StopLghtOn_B_Stat>"
  bus_selector/33 -> TrnNotInPrkChime_B_Rq/1  "<TrnNotInPrkChime_B_Rq>"
  bus_selector/34 -> WndwGlbl_D_Cmd/1  "<WndwGlbl_D_Cmd>"
  bus_selector/35 -> WrlssAcsyChrgInhbt_B_Rq/1  "<WrlssAcsyChrgInhbt_B_Rq>"

== system P702_NI_SoftECU/Output/Subsystem1/CAN_Signal/GWM/Other_GWMTx/BatteryCharge_Data2_FD1 ==
  in_port : Inport
  ChrgCrdLck_D_Falt : Terminator
  bus_selector : BusSelector  OutputSignals=ChrgCrdLck_D_Falt
  wires:
  in_port/1 -> bus_selector/1  "Subsystem1"
  bus_selector/1 -> ChrgCrdLck_D_Falt/1  "<ChrgCrdLck_D_Falt>"

== system P702_NI_SoftECU/Output/Subsystem1/CAN_Signal/GWM/Other_GWMTx/Battery_Mgmt_24V_FD1 ==
  in_port : Inport
  BattULo24Soc_Pc_Actl : Terminator
  BattULo24State_D_Qlty : Terminator
  BattULo24_Ah_DeltaRide : Terminator
  BattULo24_B_Falt : Terminator
  BattULo24_I_Actl : Terminator
  bus_selector : BusSelector  OutputSignals=BattULo24Soc_Pc_Actl,BattULo24State_D_Qlty,BattULo24_Ah_DeltaRide,BattULo24_B_Falt,BattULo24_I_Actl
  wires:
  in_port/1 -> bus_selector/1  "Subsystem1"
  bus_selector/1 -> BattULo24Soc_Pc_Actl/1  "<BattULo24Soc_Pc_Actl>"
  bus_selector/2 -> BattULo24State_D_Qlty/1  "<BattULo24State_D_Qlty>"
  bus_selector/3 -> BattULo24_Ah_DeltaRide/1  "<BattULo24_Ah_DeltaRide>"
  bus_selector/4 -> BattULo24_B_Falt/1  "<BattULo24_B_Falt>"
  bus_selector/5 -> BattULo24_I_Actl/1  "<BattULo24_I_Actl>"

== system P702_NI_SoftECU/Output/Subsystem1/CAN_Signal/GWM/Other_GWMTx/Battery_Mgmt_2_FD1 ==
  in_port : Inport
  BattULoChrg_D_Rq : Terminator
  BattULoSrvc_T_Actl : Terminator
  Batt_Crit_SoC_B : Terminator
  Batt_Lo_SoC_B : Terminator
  ChargeMode : Terminator
  EngStrtInhbt_B_RqBatt : Terminator
  IdleSpeedIncrease_El : Terminator
  PeriodicElLoad_B_Stat : Terminator
  PwSysULoFalt_D_Stat : Terminator
  Shed_Drain_Eng_Off_B : Terminator
  Shed_Feature_Group_ID : Terminator
  Shed_Level_Req : Terminator
  Shed_T_Eng_Off_B : Terminator
  ULoRgenTestMde_B_Rq : Terminator
  bus_selector : BusSelector  OutputSignals=BattULoChrg_D_Rq,BattULoSrvc_T_Actl,Batt_Crit_SoC_B,Batt_Lo_SoC_B,ChargeMode,EngStrtInhbt_B_RqBatt,IdleSpeedIncrease_El,PeriodicElLoad_B_Stat,PwSysULoFalt_D_Stat,Shed_Drain_Eng_Off_B,Shed_Feature_Group_ID,Shed_Level_Req,Shed_T_Eng_Off_B,ULoRgenTestMde_B_Rq
  wires:
  in_port/1 -> bus_selector/1  "Subsystem1"
  bus_selector/1 -> BattULoChrg_D_Rq/1  "<BattULoChrg_D_Rq>"
  bus_selector/2 -> BattULoSrvc_T_Actl/1  "<BattULoSrvc_T_Actl>"
  bus_selector/3 -> Batt_Crit_SoC_B/1  "<Batt_Crit_SoC_B>"
  bus_selector/4 -> Batt_Lo_SoC_B/1  "<Batt_Lo_SoC_B>"
  bus_selector/5 -> ChargeMode/1  "<ChargeMode>"
  bus_selector/6 -> EngStrtInhbt_B_RqBatt/1  "<EngStrtInhbt_B_RqBatt>"
  bus_selector/7 -> IdleSpeedIncrease_El/1  "<IdleSpeedIncrease_El>"
  bus_selector/8 -> PeriodicElLoad_B_Stat/1  "<PeriodicElLoad_B_Stat>"
  bus_selector/9 -> PwSysULoFalt_D_Stat/1  "<PwSysULoFalt_D_Stat>"
  bus_selector/10 -> Shed_Drain_Eng_Off_B/1  "<Shed_Drain_Eng_Off_B>"
  bus_selector/11 -> Shed_Feature_Group_ID/1  "<Shed_Feature_Group_ID>"
  bus_selector/12 -> Shed_Level_Req/1  "<Shed_Level_Req>"
  bus_selector/13 -> Shed_T_Eng_Off_B/1  "<Shed_T_Eng_Off_B>"
  bus_selector/14 -> ULoRgenTestMde_B_Rq/1  "<ULoRgenTestMde_B_Rq>"

== system P702_NI_SoftECU/Output/Subsystem1/CAN_Signal/GWM/Other_GWMTx/Battery_Mgmt_3_FD1 ==
  in_port : Inport
  BSBattQCapAh : Terminator
  BSBattQDeltaRideAh : Terminator
  BSBattSOC : Terminator
  BSFault : Terminator
  BattULo2_Te_Actl : Terminator
  BattULoChrg_URate_RqMx : Terminator
  BattULoChrg_U_RqMn : Terminator
  BattULoChrg_U_RqMx : Terminator
  BattULoState_D_Qlty : Terminator
  bus_selector : BusSelector  OutputSignals=BSBattQCapAh,BSBattQDeltaRideAh,BSBattSOC,BSFault,BattULo2_Te_Actl,BattULoChrg_URate_RqMx,BattULoChrg_U_RqMn,BattULoChrg_U_RqMx,BattULoState_D_Qlty
  wires:
  in_port/1 -> bus_selector/1  "Subsystem1"
  bus_selector/1 -> BSBattQCapAh/1  "<BSBattQCapAh>"
  bus_selector/2 -> BSBattQDeltaRideAh/1  "<BSBattQDeltaRideAh>"
  bus_selector/3 -> BSBattSOC/1  "<BSBattSOC>"
  bus_selector/4 -> BSFault/1  "<BSFault>"
  bus_selector/5 -> BattULo2_Te_Actl/1  "<BattULo2_Te_Actl>"
  bus_selector/6 -> BattULoChrg_URate_RqMx/1  "<BattULoChrg_URate_RqMx>"
  bus_selector/7 -> BattULoChrg_U_RqMn/1  "<BattULoChrg_U_RqMn>"
  bus_selector/8 -> BattULoChrg_U_RqMx/1  "<BattULoChrg_U_RqMx>"
  bus_selector/9 -> BattULoState_D_Qlty/1  "<BattULoState_D_Qlty>"

== system P702_NI_SoftECU/Output/Subsystem1/CAN_Signal/GWM/Other_GWMTx/Battery_Mgmt_4_FD1 ==
  in_port : Inport
  BattULoAuxSoc_Pc_Actl : Terminator
  BattULoAux_B_Falt : Terminator
  BattULoAux_D_Qlty : Terminator
  BattULoAux_I_Actl : Terminator
  BattULoAux_U_Actl : Terminator
  BattULoCrnkBelt_U_Pred : Terminator
  BattULoCrnkStrt_U_Pred : Terminator
  bus_selector : BusSelector  OutputSignals=BattULoAuxSoc_Pc_Actl,BattULoAux_B_Falt,BattULoAux_D_Qlty,BattULoAux_I_Actl,BattULoAux_U_Actl,BattULoCrnkBelt_U_Pred,BattULoCrnkStrt_U_Pred
  wires:
  in_port/1 -> bus_selector/1  "Subsystem1"
  bus_selector/1 -> BattULoAuxSoc_Pc_Actl/1  "<BattULoAuxSoc_Pc_Actl>"
  bus_selector/2 -> BattULoAux_B_Falt/1  "<BattULoAux_B_Falt>"
  bus_selector/3 -> BattULoAux_D_Qlty/1  "<BattULoAux_D_Qlty>"
  bus_selector/4 -> BattULoAux_I_Actl/1  "<BattULoAux_I_Actl>"
  bus_selector/5 -> BattULoAux_U_Actl/1  "<BattULoAux_U_Actl>"
  bus_selector/6 -> BattULoCrnkBelt_U_Pred/1  "<BattULoCrnkBelt_U_Pred>"
  bus_selector/7 -> BattULoCrnkStrt_U_Pred/1  "<BattULoCrnkStrt_U_Pred>"

== system P702_NI_SoftECU/Output/Subsystem1/CAN_Signal/GWM/Other_GWMTx/Battery_Traction_1_FD1 ==
  in_port : Inport
  BattTracMil_D_Rq : Terminator
  BattTracOffFst_D_Actl : Terminator
  BattTracOff_B_Actl : Terminator
  BattTrac_I_Actl : Terminator
  BattTrac_U_Actl : Terminator
  BattTrac_U_LimHi : Terminator
  BattTrac_U_LimLo : Terminator
  VehStrtInhbt_B_RqBatt : Terminator
  bus_selector : BusSelector  OutputSignals=BattTracMil_D_Rq,BattTracOffFst_D_Actl,BattTracOff_B_Actl,BattTrac_I_Actl,BattTrac_U_Actl,BattTrac_U_LimHi,BattTrac_U_LimLo,VehStrtInhbt_B_RqBatt
  wires:
  in_port/1 -> bus_selector/1  "Subsystem1"
  bus_selector/1 -> BattTracMil_D_Rq/1  "<BattTracMil_D_Rq>"
  bus_selector/2 -> BattTracOffFst_D_Actl/1  "<BattTracOffFst_D_Actl>"
  bus_selector/3 -> BattTracOff_B_Actl/1  "<BattTracOff_B_Actl>"
  bus_selector/4 -> BattTrac_I_Actl/1  "<BattTrac_I_Actl>"
  bus_selector/5 -> BattTrac_U_Actl/1  "<BattTrac_U_Actl>"
  bus_selector/6 -> BattTrac_U_LimHi/1  "<BattTrac_U_LimHi>"
  bus_selector/7 -> BattTrac_U_LimLo/1  "<BattTrac_U_LimLo>"
  bus_selector/8 -> VehStrtInhbt_B_RqBatt/1  "<VehStrtInhbt_B_RqBatt>"

== system P702_NI_SoftECU/Output/Subsystem1/CAN_Signal/GWM/Other_GWMTx/Battery_Traction_3_FD1 ==
  in_port : Inport
  BattTracClnt_Te_Actl : Terminator
  BattTracSoc_Pc_LimHi : Terminator
  BattTracSoc_Pc_LimLo : Terminator
  BattTracSoc_Pc_MnPrtct : Terminator
  BattTracSoc_Pc_MxPrtct : Terminator
  BattTracSrvcRqd_B_Rq : Terminator
  BattTracWarnLamp_B_Rq : Terminator
  bus_selector : BusSelector  OutputSignals=BattTracClnt_Te_Actl,BattTracSoc_Pc_LimHi,BattTracSoc_Pc_LimLo,BattTracSoc_Pc_MnPrtct,BattTracSoc_Pc_MxPrtct,BattTracSrvcRqd_B_Rq,BattTracWarnLamp_B_Rq
  wires:
  in_port/1 -> bus_selector/1  "Subsystem1"
  bus_selector/1 -> BattTracClnt_Te_Actl/1  "<BattTracClnt_Te_Actl>"
  bus_selector/2 -> BattTracSoc_Pc_LimHi/1  "<BattTracSoc_Pc_LimHi>"
  bus_selector/3 -> BattTracSoc_Pc_LimLo/1  "<BattTracSoc_Pc_LimLo>"
  bus_selector/4 -> BattTracSoc_Pc_MnPrtct/1  "<BattTracSoc_Pc_MnPrtct>"
  bus_selector/5 -> BattTracSoc_Pc_MxPrtct/1  "<BattTracSoc_Pc_MxPrtct>"
  bus_selector/6 -> BattTracSrvcRqd_B_Rq/1  "<BattTracSrvcRqd_B_Rq>"
  bus_selector/7 -> BattTracWarnLamp_B_Rq/1  "<BattTracWarnLamp_B_Rq>"

== system P702_NI_SoftECU/Output/Subsystem1/CAN_Signal/GWM/Other_GWMTx/Battery_Traction_4_FD1 ==
  in_port : Inport
  BattTracDiagClr_B_Rq : Terminator
  BattTracSoc2_Pc_Actl : Terminator
  BattTrac_Te_Actl : Terminator
  bus_selector : BusSelector  OutputSignals=BattTracDiagClr_B_Rq,BattTracSoc2_Pc_Actl,BattTrac_Te_Actl
  wires:
  in_port/1 -> bus_selector/1  "Subsystem1"
  bus_selector/1 -> BattTracDiagClr_B_Rq/1  "<BattTracDiagClr_B_Rq>"
  bus_selector/2 -> BattTracSoc2_Pc_Actl/1  "<BattTracSoc2_Pc_Actl>"
  bus_selector/3 -> BattTrac_Te_Actl/1  "<BattTrac_Te_Actl>"

== system P702_NI_SoftECU/Output/Subsystem1/CAN_Signal/GWM/Other_GWMTx/Battery_Traction_5_FD1 ==
  in_port : Inport
  BattTrac2_Pw_ChrgInst : Terminator
  BattTrac2_Pw_DchrgInst : Terminator
  BattTrac2_Pw_LimChrg : Terminator
  BattTrac2_Pw_LimDchrg : Terminator
  bus_selector : BusSelector  OutputSignals=BattTrac2_Pw_ChrgInst,BattTrac2_Pw_DchrgInst,BattTrac2_Pw_LimChrg,BattTrac2_Pw_LimDchrg
  wires:
  in_port/1 -> bus_selector/1  "Subsystem1"
  bus_selector/1 -> BattTrac2_Pw_ChrgInst/1  "<BattTrac2_Pw_ChrgInst>"
  bus_selector/2 -> BattTrac2_Pw_DchrgInst/1  "<BattTrac2_Pw_DchrgInst>"
  bus_selector/3 -> BattTrac2_Pw_LimChrg/1  "<BattTrac2_Pw_LimChrg>"
  bus_selector/4 -> BattTrac2_Pw_LimDchrg/1  "<BattTrac2_Pw_LimDchrg>"

== system P702_NI_SoftECU/Output/Subsystem1/CAN_Signal/GWM/Other_GWMTx/Battery_Traction_6_FD1 ==
  in_port : Inport
  BattTracClntPmp_D_Stat : Terminator
  BattTracCnnct_D_Cmd : Terminator
  BattTracDcdcDis_B_Rq : Terminator
  BattTracDelta_Te_Actl : Terminator
  BattTracHvilOpen_B_Stat : Terminator
  HtrnClntPump_D_Stat : Terminator
  bus_selector : BusSelector  OutputSignals=BattTracClntPmp_D_Stat,BattTracCnnct_D_Cmd,BattTracDcdcDis_B_Rq,BattTracDelta_Te_Actl,BattTracHvilOpen_B_Stat,HtrnClntPump_D_Stat
  wires:
  in_port/1 -> bus_selector/1  "Subsystem1"
  bus_selector/1 -> BattTracClntPmp_D_Stat/1  "<BattTracClntPmp_D_Stat>"
  bus_selector/2 -> BattTracCnnct_D_Cmd/1  "<BattTracCnnct_D_Cmd>"
  bus_selector/3 -> BattTracDcdcDis_B_Rq/1  "<BattTracDcdcDis_B_Rq>"
  bus_selector/4 -> BattTracDelta_Te_Actl/1  "<BattTracDelta_Te_Actl>"
  bus_selector/5 -> BattTracHvilOpen_B_Stat/1  "<BattTracHvilOpen_B_Stat>"
  bus_selector/6 -> HtrnClntPump_D_Stat/1  "<HtrnClntPump_D_Stat>"

== system P702_NI_SoftECU/Output/Subsystem1/CAN_Signal/GWM/Other_GWMTx/BodyInfo_3_FD1 ==
  in_port : Inport
  Backlit_LED_Status : Terminator
  BodySrvcRqd_B_Rq : Terminator
  CrashEvnt_D_Stat : Terminator
  Day_Night_Status : Terminator
  Delay_Accy : Terminator
  DimmingLvlEvnt_No_Actl : Terminator
  Dimming_Lvl : Terminator
  DrStatDrvErrCnt_B_Stat : Terminator
  DrStatDrv_B_Actl : Terminator
  DrStatHood_B_Actl : Terminator
  DrStatInnrTgate_B_Actl : Terminator
  DrStatPsngr_B_Actl : Terminator
  DrStatRl_B_Actl : Terminator
  DrStatRr_B_Actl : Terminator
  DrStatTgate_B_Actl : Terminator
  FogLghtFrontOn_B_Stat : Terminator
  FogLghtRearOn_B_Stat : Terminator
  FuelPmpInhbt_B_Stat : Terminator
  IgnKeyType_D_Actl : Terminator
  Ignition_Status : Terminator
  Key_In_Ignition_Stat : Terminator
  LifeCycMde_D_Actl : Terminator
  Litval : Terminator
  Parklamp_Status : Terminator
  PrkBrkActv_B_Actl : Terminator
  Remote_Start_Status : Terminator
  TurnLghtLeftOn_B_Stat : Terminator
  TurnLghtLeft_D_Rq : Terminator
  TurnLghtRightOn_B_Stat : Terminator
  TurnLghtRight_D_Rq : Terminator
  ValetMode_D_Mem : Terminator
  bus_selector : BusSelector  OutputSignals=Backlit_LED_Status,BodySrvcRqd_B_Rq,CrashEvnt_D_Stat,Day_Night_Status,Delay_Accy,DimmingLvlEvnt_No_Actl,Dimming_Lvl,DrStatDrvErrCnt_B_Stat,DrStatDrv_B_Actl,DrStatHood_B_Actl,DrStatInnrTgate_B_Actl,DrStatPsngr_B_Actl,DrStatRl_B_Actl,DrStatRr_B_Actl,DrStatTgate_B_Actl,FogLghtFrontOn_B_Stat,FogLghtRearOn_B_Stat,FuelPmpInhbt_B_Stat,IgnKeyType_D_Actl,Ignition_Status,Key_In_Ignition_Stat,LifeCycMde_D_Actl,Litval,Parklamp_Status,PrkBrkActv_B_Actl,Remote_Start_Status,TurnLghtLeftOn_B_Stat,TurnLghtLeft_D_Rq,TurnLghtRightOn_B_Stat,TurnLghtRight_D_Rq,ValetMode_D_Mem
  wires:
  in_port/1 -> bus_selector/1  "Subsystem1"
  bus_selector/1 -> Backlit_LED_Status/1  "<Backlit_LED_Status>"
  bus_selector/2 -> BodySrvcRqd_B_Rq/1  "<BodySrvcRqd_B_Rq>"
  bus_selector/3 -> CrashEvnt_D_Stat/1  "<CrashEvnt_D_Stat>"
  bus_selector/4 -> Day_Night_Status/1  "<Day_Night_Status>"
  bus_selector/5 -> Delay_Accy/1  "<Delay_Accy>"
  bus_selector/6 -> DimmingLvlEvnt_No_Actl/1  "<DimmingLvlEvnt_No_Actl>"
  bus_selector/7 -> Dimming_Lvl/1  "<Dimming_Lvl>"
  bus_selector/8 -> DrStatDrvErrCnt_B_Stat/1  "<DrStatDrvErrCnt_B_Stat>"
  bus_selector/9 -> DrStatDrv_B_Actl/1  "<DrStatDrv_B_Actl>"
  bus_selector/10 -> DrStatHood_B_Actl/1  "<DrStatHood_B_Actl>"
  bus_selector/11 -> DrStatInnrTgate_B_Actl/1  "<DrStatInnrTgate_B_Actl>"
  bus_selector/12 -> DrStatPsngr_B_Actl/1  "<DrStatPsngr_B_Actl>"
  bus_selector/13 -> DrStatRl_B_Actl/1  "<DrStatRl_B_Actl>"
  bus_selector/14 -> DrStatRr_B_Actl/1  "<DrStatRr_B_Actl>"
  bus_selector/15 -> DrStatTgate_B_Actl/1  "<DrStatTgate_B_Actl>"
  bus_selector/16 -> FogLghtFrontOn_B_Stat/1  "<FogLghtFrontOn_B_Stat>"
  bus_selector/17 -> FogLghtRearOn_B_Stat/1  "<FogLghtRearOn_B_Stat>"
  bus_selector/18 -> FuelPmpInhbt_B_Stat/1  "<FuelPmpInhbt_B_Stat>"
  bus_selector/19 -> IgnKeyType_D_Actl/1  "<IgnKeyType_D_Actl>"
  bus_selector/20 -> Ignition_Status/1  "<Ignition_Status>"
  bus_selector/21 -> Key_In_Ignition_Stat/1  "<Key_In_Ignition_Stat>"
  bus_selector/22 -> LifeCycMde_D_Actl/1  "<LifeCycMde_D_Actl>"
  bus_selector/23 -> Litval/1  "<Litval>"
  bus_selector/24 -> Parklamp_Status/1  "<Parklamp_Status>"
  bus_selector/25 -> PrkBrkActv_B_Actl/1  "<PrkBrkActv_B_Actl>"
  bus_selector/26 -> Remote_Start_Status/1  "<Remote_Start_Status>"
  bus_selector/27 -> TurnLghtLeftOn_B_Stat/1  "<TurnLghtLeftOn_B_Stat>"
  bus_selector/28 -> TurnLghtLeft_D_Rq/1  "<TurnLghtLeft_D_Rq>"
  bus_selector/29 -> TurnLghtRightOn_B_Stat/1  "<TurnLghtRightOn_B_Stat>"
  bus_selector/30 -> TurnLghtRight_D_Rq/1  "<TurnLghtRight_D_Rq>"
  bus_selector/31 -> ValetMode_D_Mem/1  "<ValetMode_D_Mem>"

== system P702_NI_SoftECU/Output/Subsystem1/CAN_Signal/GWM/Other_GWMTx/Body_Info_10_FD1 ==
  in_port : Inport
  GenericSwtch1_No_Actl : Terminator
  GenericSwtch2_No_Actl : Terminator
  GenericSwtch3_No_Actl : Terminator
  bus_selector : BusSelector  OutputSignals=GenericSwtch1_No_Actl,GenericSwtch2_No_Actl,GenericSwtch3_No_Actl
  wires:
  in_port/1 -> bus_selector/1  "Subsystem1"
  bus_selector/1 -> GenericSwtch1_No_Actl/1  "<GenericSwtch1_No_Actl>"
  bus_selector/2 -> GenericSwtch2_No_Actl/1  "<GenericSwtch2_No_Actl>"
  bus_selector/3 -> GenericSwtch3_No_Actl/1  "<GenericSwtch3_No_Actl>"

== system P702_NI_SoftECU/Output/Subsystem1/CAN_Signal/GWM/Other_GWMTx/Body_Info_4_FD1 ==
  in_port : Inport
  BattULo_I_Actl : Terminator
  BattULo_U_Actl : Terminator
  BrkTrnShifLck_B_Stat : Terminator
  DcacElPw_D_Rq : Terminator
  DriverCrankingReq : Terminator
  EngOff_T_Actl : Terminator
  FuelPumpPwr_D_Stat : Terminator
  PrkLckCtlAvail_T_Stat : Terminator
  PrkLckCtlMsgTxt_D_Rq : Terminator
  PrkLckCtlTow_B_Enbl : Terminator
  PrkLckCtlUnlck_D_Stat : Terminator
  PrkLckCtl_B_Enbl : Terminator
  PtLatchActv_B_RqBcm : Terminator
  ReFuelSwtchStat_D_Actl : Terminator
  bus_selector : BusSelector  OutputSignals=BattULo_I_Actl,BattULo_U_Actl,BrkTrnShifLck_B_Stat,DcacElPw_D_Rq,DriverCrankingReq,EngOff_T_Actl,FuelPumpPwr_D_Stat,PrkLckCtlAvail_T_Stat,PrkLckCtlMsgTxt_D_Rq,PrkLckCtlTow_B_Enbl,PrkLckCtlUnlck_D_Stat,PrkLckCtl_B_Enbl,PtLatchActv_B_RqBcm,ReFuelSwtchStat_D_Actl,immoSecureIdleMode
  immoSecureIdleMode : Terminator
  wires:
  in_port/1 -> bus_selector/1  "Subsystem1"
  bus_selector/1 -> BattULo_I_Actl/1  "<BattULo_I_Actl>"
  bus_selector/2 -> BattULo_U_Actl/1  "<BattULo_U_Actl>"
  bus_selector/3 -> BrkTrnShifLck_B_Stat/1  "<BrkTrnShifLck_B_Stat>"
  bus_selector/4 -> DcacElPw_D_Rq/1  "<DcacElPw_D_Rq>"
  bus_selector/5 -> DriverCrankingReq/1  "<DriverCrankingReq>"
  bus_selector/6 -> EngOff_T_Actl/1  "<EngOff_T_Actl>"
  bus_selector/7 -> FuelPumpPwr_D_Stat/1  "<FuelPumpPwr_D_Stat>"
  bus_selector/8 -> PrkLckCtlAvail_T_Stat/1  "<PrkLckCtlAvail_T_Stat>"
  bus_selector/9 -> PrkLckCtlMsgTxt_D_Rq/1  "<PrkLckCtlMsgTxt_D_Rq>"
  bus_selector/10 -> PrkLckCtlTow_B_Enbl/1  "<PrkLckCtlTow_B_Enbl>"
  bus_selector/11 -> PrkLckCtlUnlck_D_Stat/1  "<PrkLckCtlUnlck_D_Stat>"
  bus_selector/12 -> PrkLckCtl_B_Enbl/1  "<PrkLckCtl_B_Enbl>"
  bus_selector/13 -> PtLatchActv_B_RqBcm/1  "<PtLatchActv_B_RqBcm>"
  bus_selector/14 -> ReFuelSwtchStat_D_Actl/1  "<ReFuelSwtchStat_D_Actl>"
  bus_selector/15 -> immoSecureIdleMode/1  "<immoSecureIdleMode>"

== system P702_NI_SoftECU/Output/Subsystem1/CAN_Signal/GWM/Other_GWMTx/Body_Info_6_FD1 ==
  in_port : Inport
  DrLatchMsgTxt_D_Rq : Terminator
  ElPwPoint_D_Rq : Terminator
  HeadLghtHiPrmsn_D_Stat : Terminator
  IgnPsswrdDsply_B_Rq : Terminator
  KeyAdmnTot_No_Cnt : Terminator
  KeyMykeyTot_No_Cnt : Terminator
  Keycode_Status : Terminator
  PEBackupSlot_Stats : Terminator
  PoliceIdlMde_D_Stat : Terminator
  PrmtrAlrmEvnt_D_Stat : Terminator
  PrsnlDevcChrgEnbl_B_Rq : Terminator
  SecurityMsgTxt_D_Rq : Terminator
  SteWhlLckMsgTxt_D_Rq : Terminator
  TracKeyMde_D_Stat : Terminator
  bus_selector : BusSelector  OutputSignals=DrLatchMsgTxt_D_Rq,ElPwPoint_D_Rq,HeadLghtHiPrmsn_D_Stat,IgnPsswrdDsply_B_Rq,KeyAdmnTot_No_Cnt,KeyMykeyTot_No_Cnt,Keycode_Status,PEBackupSlot_Stats,PoliceIdlMde_D_Stat,PrmtrAlrmEvnt_D_Stat,PrsnlDevcChrgEnbl_B_Rq,SecurityMsgTxt_D_Rq,SteWhlLckMsgTxt_D_Rq,TracKeyMde_D_Stat,immoMsgTxt_D_Rq
  immoMsgTxt_D_Rq : Terminator
  wires:
  in_port/1 -> bus_selector/1  "Subsystem1"
  bus_selector/1 -> DrLatchMsgTxt_D_Rq/1  "<DrLatchMsgTxt_D_Rq>"
  bus_selector/2 -> ElPwPoint_D_Rq/1  "<ElPwPoint_D_Rq>"
  bus_selector/3 -> HeadLghtHiPrmsn_D_Stat/1  "<HeadLghtHiPrmsn_D_Stat>"
  bus_selector/4 -> IgnPsswrdDsply_B_Rq/1  "<IgnPsswrdDsply_B_Rq>"
  bus_selector/5 -> KeyAdmnTot_No_Cnt/1  "<KeyAdmnTot_No_Cnt>"
  bus_selector/6 -> KeyMykeyTot_No_Cnt/1  "<KeyMykeyTot_No_Cnt>"
  bus_selector/7 -> Keycode_Status/1  "<Keycode_Status>"
  bus_selector/8 -> PEBackupSlot_Stats/1  "<PEBackupSlot_Stats>"
  bus_selector/9 -> PoliceIdlMde_D_Stat/1  "<PoliceIdlMde_D_Stat>"
  bus_selector/10 -> PrmtrAlrmEvnt_D_Stat/1  "<PrmtrAlrmEvnt_D_Stat>"
  bus_selector/11 -> PrsnlDevcChrgEnbl_B_Rq/1  "<PrsnlDevcChrgEnbl_B_Rq>"
  bus_selector/12 -> SecurityMsgTxt_D_Rq/1  "<SecurityMsgTxt_D_Rq>"
  bus_selector/13 -> SteWhlLckMsgTxt_D_Rq/1  "<SteWhlLckMsgTxt_D_Rq>"
  bus_selector/14 -> TracKeyMde_D_Stat/1  "<TracKeyMde_D_Stat>"
  bus_selector/15 -> immoMsgTxt_D_Rq/1  "<immoMsgTxt_D_Rq>"

== system P702_NI_SoftECU/Output/Subsystem1/CAN_Signal/GWM/Other_GWMTx/Body_Info_8_FD1 ==
  in_port : Inport
  ChrgCordLck_B_Stat : Terminator
  ChrgCordResp1_No_Actl : Terminator
  ChrgCordResp2_No_Actl : Terminator
  WakeAlarm0_D_Stat : Terminator
  WakeAlarm1_D_Stat : Terminator
  WakeAlarm2_D_Stat : Terminator
  WakeAlarm3_D_Stat : Terminator
  bus_selector : BusSelector  OutputSignals=ChrgCordLck_B_Stat,ChrgCordResp1_No_Actl,ChrgCordResp2_No_Actl,WakeAlarm0_D_Stat,WakeAlarm1_D_Stat,WakeAlarm2_D_Stat,WakeAlarm3_D_Stat
  wires:
  in_port/1 -> bus_selector/1  "Subsystem1"
  bus_selector/1 -> ChrgCordLck_B_Stat/1  "<ChrgCordLck_B_Stat>"
  bus_selector/2 -> ChrgCordResp1_No_Actl/1  "<ChrgCordResp1_No_Actl>"
  bus_selector/3 -> ChrgCordResp2_No_Actl/1  "<ChrgCordResp2_No_Actl>"
  bus_selector/4 -> WakeAlarm0_D_Stat/1  "<WakeAlarm0_D_Stat>"
  bus_selector/5 -> WakeAlarm1_D_Stat/1  "<WakeAlarm1_D_Stat>"
  bus_selector/6 -> WakeAlarm2_D_Stat/1  "<WakeAlarm2_D_Stat>"
  bus_selector/7 -> WakeAlarm3_D_Stat/1  "<WakeAlarm3_D_Stat>"

== system P702_NI_SoftECU/Output/Subsystem1/CAN_Signal/GWM/Other_GWMTx/Body_Info_9_FD1 ==
  in_port : Inport
  AdvStrt_D_Stat : Terminator
  CrnkInhbt_B_Stat : Terminator
  CrnkInhbt_No_Cnt : Terminator
  CrnkInhbt_No_Cs : Terminator
  DrvInCtl_B_Stat : Terminator
  EngStrtActv_B_Stat : Terminator
  EngStrt_B_Rq : Terminator
  IgnPreOffActv_B_Stat : Terminator
  StrtrMtrCtlDStat_No_Cs : Terminator
  VehOnSrc_D_Stat : Terminator
  bus_selector : BusSelector  OutputSignals=AdvStrt_D_Stat,CrnkInhbt_B_Stat,CrnkInhbt_No_Cnt,CrnkInhbt_No_Cs,DrvInCtl_B_Stat,EngStrtActv_B_Stat,EngStrt_B_Rq,IgnPreOffActv_B_Stat,StrtrMtrCtlDStat_No_Cs,VehOnSrc_D_Stat
  wires:
  in_port/1 -> bus_selector/1  "Subsystem1"
  bus_selector/1 -> AdvStrt_D_Stat/1  "<AdvStrt_D_Stat>"
  bus_selector/2 -> CrnkInhbt_B_Stat/1  "<CrnkInhbt_B_Stat>"
  bus_selector/3 -> CrnkInhbt_No_Cnt/1  "<CrnkInhbt_No_Cnt>"
  bus_selector/4 -> CrnkInhbt_No_Cs/1  "<CrnkInhbt_No_Cs>"
  bus_selector/5 -> DrvInCtl_B_Stat/1  "<DrvInCtl_B_Stat>"
  bus_selector/6 -> EngStrtActv_B_Stat/1  "<EngStrtActv_B_Stat>"
  bus_selector/7 -> EngStrt_B_Rq/1  "<EngStrt_B_Rq>"
  bus_selector/8 -> IgnPreOffActv_B_Stat/1  "<IgnPreOffActv_B_Stat>"
  bus_selector/9 -> StrtrMtrCtlDStat_No_Cs/1  "<StrtrMtrCtlDStat_No_Cs>"
  bus_selector/10 -> VehOnSrc_D_Stat/1  "<VehOnSrc_D_Stat>"
